simulink model "MAGNETOMETER"  (R2024b)
settings: Solver=ode8  StartTime=0.0  StopTime=10.0  FixedStep=0.01  RelTol=1e-3
undefined symbols (not defined in the file or in its folder): sensor
settings Model: Creator=eleon  LastModifiedBy=eleon

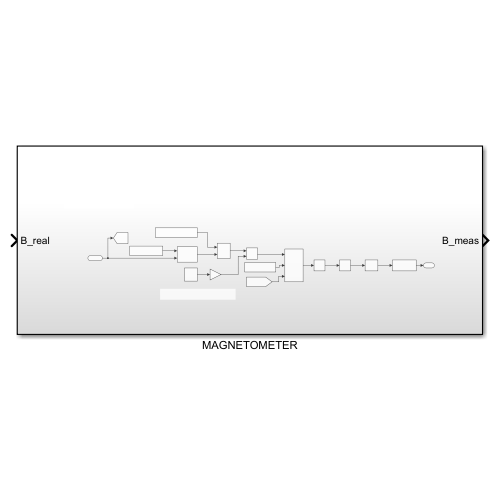
[thumbnail: Simulink's stored preview of the top-level diagram]
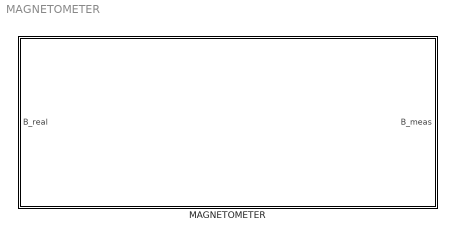
== system MAGNETOMETER ==
  MAGNETOMETER : Subsystem

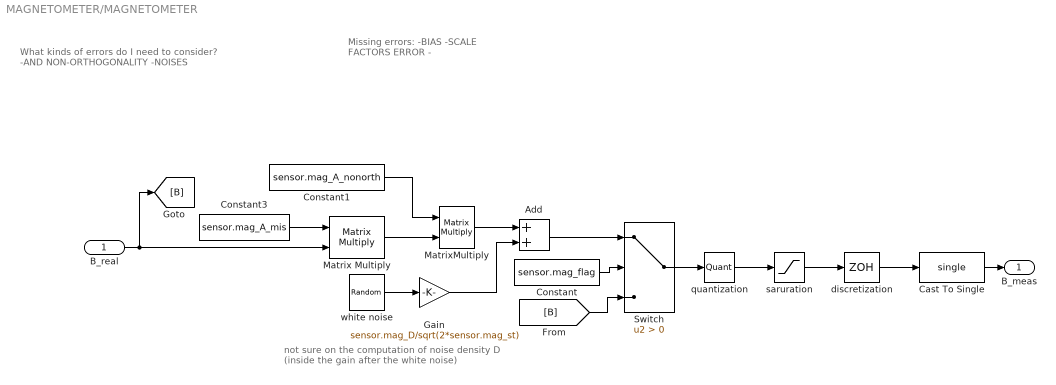
== system MAGNETOMETER/MAGNETOMETER ==
  note: not sure on the computation of noise density D (inside the gain after the white noise)
  note: Missing errors:
      | -BIAS
      | -SCALE FACTORS ERROR
      | -
  note: What kinds of errors do I need to consider?
      | -AND NON-ORTHOGONALITY
      | -NOISES
  B_real : Inport
  Add : Sum
  Cast To Single : DataTypeConversion  OutDataTypeStr=single  SaturateOnIntegerOverflow=off  RndMeth=Floor
  Constant : Constant  Value=sensor.mag_flag
  Constant1 : Constant  Value=sensor.mag_A_nonorth
  Constant3 : Constant  Value=sensor.mag_A_mis
  Gain : Gain  Gain=sensor.mag_D/sqrt(2*sensor.mag_st)
  Matrix Multiply : Product  Multiplication=Matrix(*)
  MatrixMultiply : Product  Multiplication=Matrix(*)
  Switch : Switch  Criteria=u2 > Threshold  SaturateOnIntegerOverflow=off  InputSameDT=off
  "discretization " : ZeroOrderHold  SampleTime=sensor.mag_st
  quantization : Quantizer  QuantizationInterval=sensor.mag_quant
  saruration : Saturate  UpperLimit=sensor.mag_sat(1,1)  LowerLimit=sensor.mag_sat(1,2)
  white noise : RandomNumber  SampleTime=sensor.mag_st
  B_meas : Outport
  wires:
  B_real/1 -> [B], Matrix Multiply/2
  [B] -> Switch/3
  Constant/1 -> Switch/2
  Switch/1 -> quantization/1
  "discretization "/1 -> Cast To Single/1
  white noise/1 -> Gain/1
  saruration/1 -> "discretization "/1
  quantization/1 -> saruration/1
  Gain/1 -> Add/2
  Constant3/1 -> Matrix Multiply/1
  Matrix Multiply/1 -> MatrixMultiply/2
  Constant1/1 -> MatrixMultiply/1
  MatrixMultiply/1 -> Add/1
  Cast To Single/1 -> B_meas/1
  Add/1 -> Switch/1
